simulink model "Rendezvous_sim"  (R2024b)
settings: Solver=VariableStepAuto  StartTime=0.0  StopTime=5e4  MaxStep=50  RelTol=1e-6
undefined symbols (not defined in the file or in its folder): target
settings Model: Creator=cpero  LastModifiedBy=cpero

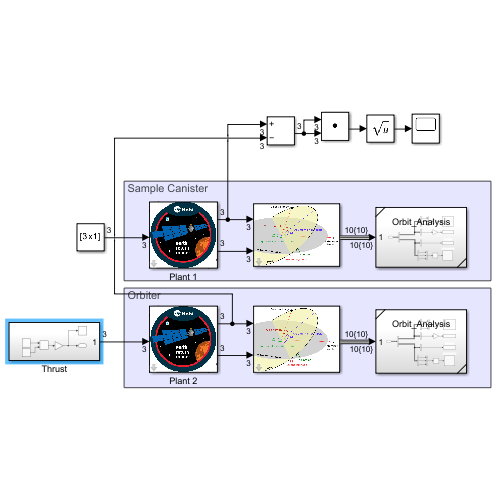
[thumbnail: Simulink's stored preview of the top-level diagram]
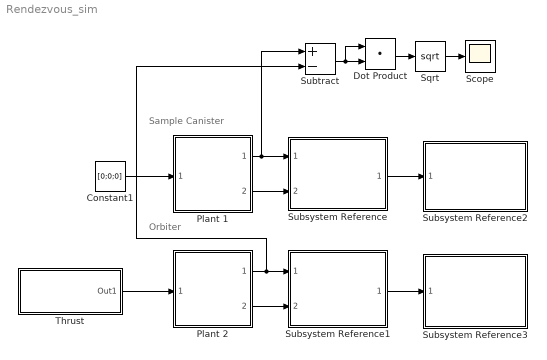
== system Rendezvous_sim ==
  note: Orbiter
  note: Sample Canister
  Constant1 : Constant  Value=[0;0;0]
  Dot Product : DotProduct  OutDataTypeStr=Inherit: Inherit via internal rule
  Plant 1 : Subsystem  ReferencedSubsystem=Plant  setup=rendezvous_data.canister_initial  switch_time=0  mu=Mars_planet.mu
  Plant 2 : Subsystem  ReferencedSubsystem=Plant  setup=rendezvous_data.orbiter_initial  switch_time=0  mu=Mars_planet.mu
  Scope : Scope
  Sqrt : Sqrt
  Subsystem Reference : Subsystem  ReferencedSubsystem=Orbit_Calculations  mu=Mars_planet.mu
  Subsystem Reference1 : Subsystem  ReferencedSubsystem=Orbit_Calculations  mu=Mars_planet.mu
  Subsystem Reference2 : Subsystem  ReferencedSubsystem=Orbit_Analysis
  Subsystem Reference3 : Subsystem  ReferencedSubsystem=Orbit_Analysis
  Subtract : Sum  Inputs=+-
  Thrust : Subsystem
  wires:
  Plant 1/1 -> Subtract/1, Subsystem Reference/1
  Plant 2/2 -> Subsystem Reference1/2
  Plant 1/2 -> Subsystem Reference/2
  Thrust/1(Out1) -> Plant 2/1
  Constant1/1 -> Plant 1/1
  Subsystem Reference/1 -> Subsystem Reference2/1
  Subsystem Reference1/1 -> Subsystem Reference3/1
  Plant 2/1 -> Subtract/2, Subsystem Reference1/1
  Subtract/1 -> Dot Product/1, Dot Product/2
  Dot Product/1 -> Sqrt/1
  Sqrt/1 -> Scope/1

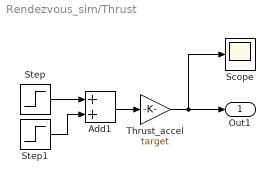
== system Rendezvous_sim/Thrust ==
  Add1 : Sum
  Scope : Scope
  Step : Step  SampleTime=0
  Step1 : Step  Time=1 + 1  After=-1  SampleTime=0
  Thrust_accel : Gain  Gain=target
  Out1 : Outport
  wires:
  Add1/1 -> Thrust_accel/1
  Thrust_accel/1 -> Out1/1, Scope/1
  Step1/1 -> Add1/2
  Step/1 -> Add1/1
